simulink model "MatlabFunction_TestGen_dot4"  (R2017b)
settings: Solver=FixedStepDiscrete  StartTime=0.0  StopTime=10.0  RelTol=1e-3
settings Model: Creator=ktrinh  LastModifiedBy=ktrinh
settings DebuggingCC: ParameterOverflowMsg=none

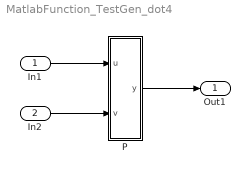
== system MatlabFunction_TestGen_dot4 ==
  In1 : Inport  OutDataTypeStr=single  PortDimensions=[2,3]
  In2 : Inport  Port=2  OutDataTypeStr=single  PortDimensions=[2,3]
  P : MATLAB Function  TreatAsAtomicUnit=on
  Out1 : Outport
  wires:
  In1/1 -> P/1(u)
  In2/1 -> P/2(v)
  P/1(y) -> Out1/1

== matlab function MatlabFunction_TestGen_dot4/P ==
  data: u input; y output; v input
function y = fcn(u, v)
y = dot(u, v);
